simulink model "laby2_2"  (R2024b)
settings: Solver=VariableStepAuto  StartTime=0.0  StopTime=250.0  RelTol=1e-3
settings Model: Creator=Jakub Janiczuk  LastModifiedBy=Jakub Janiczuk

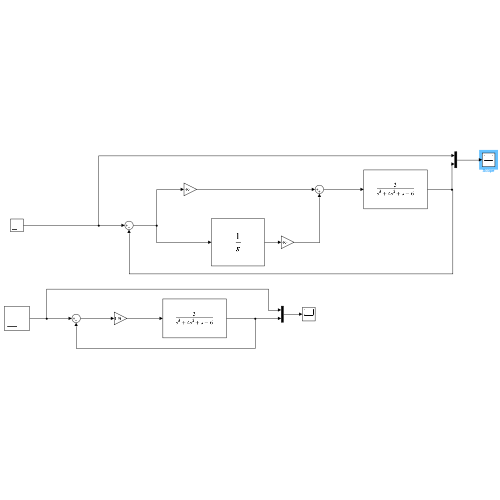
[thumbnail: Simulink's stored preview of the top-level diagram]
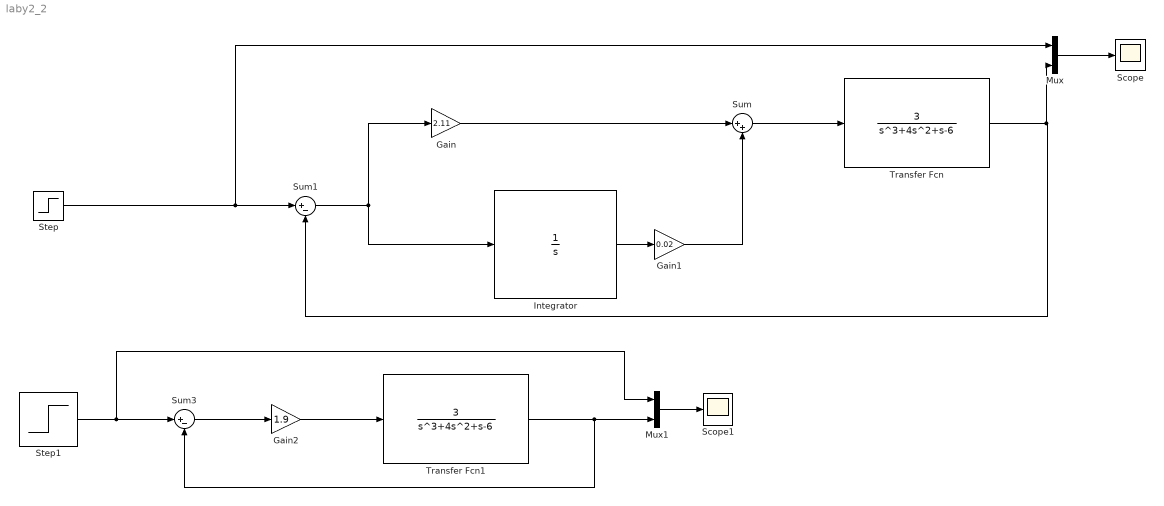
== system laby2_2 ==
  Gain : Gain  Gain=2.11
  Gain1 : Gain  Gain=0.02
  Gain2 : Gain  Gain=1.9
  Integrator : Integrator  InitialCondition=1
  Mux : Mux  Inputs=2
  Mux1 : Mux  Inputs=2
  Scope : Scope
  Scope1 : Scope
  Step : Step  SampleTime=0
  Step1 : Step  SampleTime=0
  Sum : Sum  Inputs=|++
  Sum1 : Sum  Inputs=|+-
  Sum3 : Sum  Inputs=|+-
  Transfer Fcn : TransferFcn  Numerator=[3]  Denominator=[1 4 1 -6 ]
  Transfer Fcn1 : TransferFcn  Numerator=[3]  Denominator=[1 4 1 -6 ]
  wires:
  Step/1 -> Mux/1, Sum1/1
  Sum/1 -> Transfer Fcn/1
  Transfer Fcn/1 -> Mux/2, Sum1/2
  Sum1/1 -> Gain/1, Integrator/1
  Gain/1 -> Sum/1
  Integrator/1 -> Gain1/1
  Gain1/1 -> Sum/2
  Mux/1 -> Scope/1
  Gain2/1 -> Transfer Fcn1/1
  Step1/1 -> Mux1/1, Sum3/1
  Transfer Fcn1/1 -> Sum3/2, Mux1/2
  Sum3/1 -> Gain2/1
  Mux1/1 -> Scope1/1
